simulink model "BaseMotion"  (R2022b)
settings: Solver=VariableStepAuto  StartTime=0.0  StopTime=10.0  RelTol=1e-3
libraries: roblocks x4
settings Model: Creator=Artem  LastModifiedBy=iarte

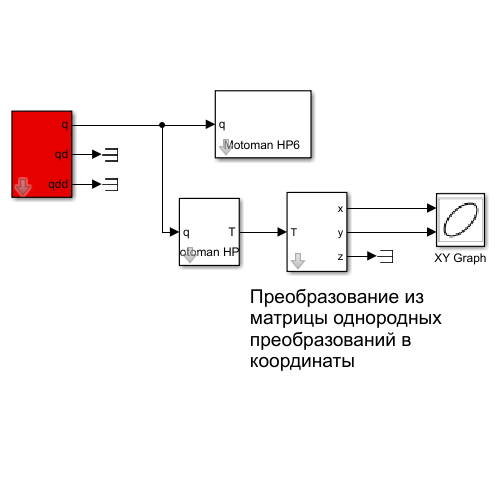
[thumbnail: Simulink's stored preview of the top-level diagram]
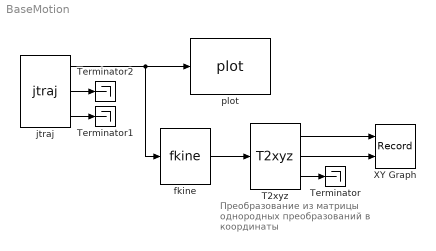
== system BaseMotion ==
  note: Преобразование из матрицы однородных преобразований в координаты
  T2xyz : roblocks/Toolbox/T2xyz
  Terminator : Terminator
  Terminator1 : Terminator
  Terminator2 : Terminator
  XY Graph : Record  FileSettingsInternal="{\"entries\":[{\"content\":{\"excelSettings\":{\"content\":{},\"type\":\"Streamout.ExcelSettings\"}},\"type\":\"Streamout.FileSettingStorage\",\"uuid\":\"320995ab-50ca-47a6-835d-657ee2e82bbb\"}],\"packageUris\":[\"http://schema.mathworks.com/mf0/streamout_blocks/R2020a\"],\"version\":\"1.0\"}"  Layout=[1 1]  SignalsInternal="{\"entries\":[{\"content\":{\"signals\":[{\"content\":{\"blockPath\":[\"lr2/XY Graph\"],\"channel\":[],\"dimensions\":[1],\"domain\":\"lr2/XY Graph\",\"lineColor\":\"#a2142f\",\"plots\":[1],\"port\":1,\"sid\":[\"\"],\"signalID\":117,\"signalName\":\"T2xyz:1\"},\"type\":\"RecordBlkView.Signal\",\"uuid\":\"cb58e3d4-ba62-4844-acf9-b532e0bf00de\"},{\"content\":{\"blockPath\":[\"lr2/XY Graph\"],\"channel\":[],\"dimensions\":[1],\"domain\":\"lr2/XY Graph\",\"lineColor\":\"#139fff\",\"plots\":[1],\"port\":2,\"sid\":[\"\"],\"signalID\":121,\"signalName\":\"T2xyz:2\"},\"type\":\"RecordBlkView.Signal\",\"uuid\":\"dc694c10-232d-46e5-9600-0cb1e34927e4\"}]},\"type\":\"RecordBlkView.InputSignals\",\"uuid\":\"5149e04e-9650-4c10-a57e-e2ab91be6986\"}],\"packageUris\":[\"http://schema.mathworks.com/mf0/streamout_blocks/R2020a\"],\"version\":\"1.0\"}"  VisualizationBindings="{\"xyplotplugin\":{\"info\":[{\"series\":[{\"bindingParametersList\":[{\"parameter\":\"X-Axis\",\"signalID\":117,\"signalName\":\"T2xyz:1\"},{\"parameter\":\"Y-Axis\",\"signalID\":121,\"signalName\":\"T2xyz:2\"}],\"seriesID\":50130}],\"subplotID\":1}]}}"  CompatibilityTag=XY  st=-1
  fkine : roblocks/Arm/fkine  robot=hp6
  jtraj : roblocks/Toolbox/jtraj  q0=[0 0 0 0 0 0]  qf=[0.6747 -2.2248 -0.8732 1.3986 0.9150 -2.8637]  tmax=5  ts=0.02
  plot : roblocks/Arm/plot  robot=hp6  fps=25  holdplot=on
  wires:
  jtraj/1 -> plot/1, fkine/1
  T2xyz/2 -> XY Graph/2
  jtraj/2 -> Terminator2/1
  T2xyz/1 -> XY Graph/1
  jtraj/3 -> Terminator1/1
  T2xyz/3 -> Terminator/1
  fkine/1 -> T2xyz/1
